simulink subsystem "linear_slope_score"  (R2020b)
settings: Solver=VariableStepAuto  StartTime=0.0  StopTime=10.0  RelTol=1e-3
settings Model: Creator=RH  LastModifiedBy=Marco

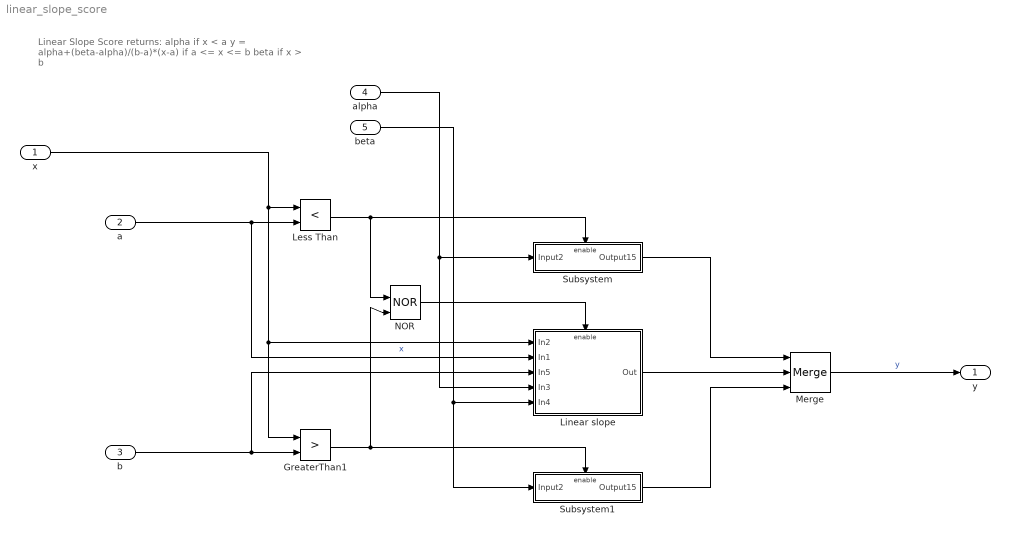
== system linear_slope_score ==
  note: Linear Slope Score
      | returns:
      |
      | alpha if x < a
      | y = alpha+(beta-alpha)/(b-a)*(x-a) if a <= x <= b
      | beta if x > b
  x : Inport
  a : Inport  Port=2
  b : Inport  Port=3
  alpha : Inport  Port=4
  beta : Inport  Port=5
  GreaterThan1 : RelationalOperator  Operator=>  OutDataTypeStr=boolean  RndMeth=Simplest
  Less Than : RelationalOperator  Operator=<  OutDataTypeStr=boolean  RndMeth=Simplest
  Linear slope : Subsystem
  Merge : Merge  Inputs=3
  NOR : Logic  Operator=NOR  IconShape=distinctive  AllPortsSameDT=off  OutDataTypeStr=boolean
  Subsystem : Subsystem
  Subsystem1 : Subsystem
  y : Outport
  wires:
  b/1 -> Linear slope/3(In5), GreaterThan1/2
  Less Than/1 -> NOR/1, Subsystem/Enable
  x/1 -> Linear slope/1(In2), GreaterThan1/1, Less Than/1  "x"
  beta/1 -> Linear slope/5(In4), Subsystem1/1(Input2)
  alpha/1 -> Subsystem/1(Input2), Linear slope/4(In3)
  Subsystem/1(Output15) -> Merge/1
  GreaterThan1/1 -> NOR/2, Subsystem1/Enable
  a/1 -> Linear slope/2(In1), Less Than/2
  NOR/1 -> Linear slope/Enable
  Subsystem1/1(Output15) -> Merge/3
  Linear slope/1(Out) -> Merge/2
  Merge/1 -> y/1  "y"

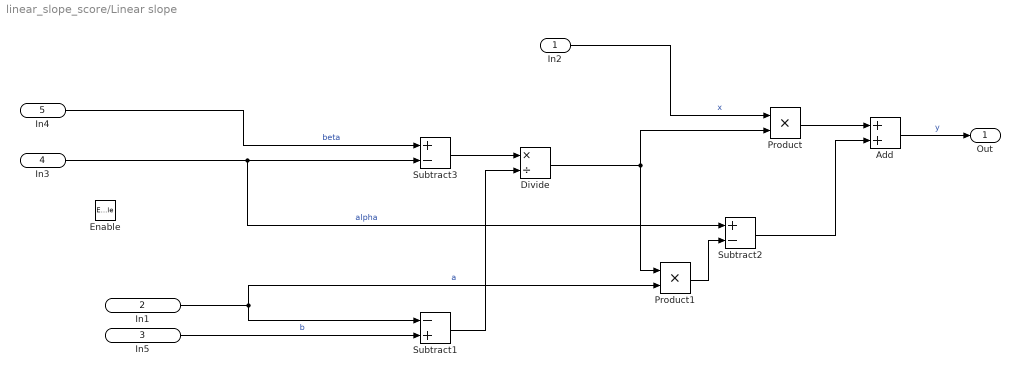
== system linear_slope_score/Linear slope ==
  In2 : Inport
  In1 : Inport  Port=2
  In5 : Inport  Port=3
  In3 : Inport  Port=4  Unit=1
  In4 : Inport  Port=5  Unit=1
  Enable : EnablePort
  Add : Sum
  Divide : Product  Inputs=*/
  Product : Product
  Product1 : Product
  Subtract1 : Sum  Inputs=-+
  Subtract2 : Sum  Inputs=+-
  Subtract3 : Sum  Inputs=+-
  Out : Outport  Unit=1
  wires:
  In4/1 -> Subtract3/1  "beta"
  Subtract2/1 -> Add/2
  Product1/1 -> Subtract2/2
  Add/1 -> Out/1  "y"
  Product/1 -> Add/1
  Divide/1 -> Product1/1, Product/2
  Subtract1/1 -> Divide/2
  In5/1 -> Subtract1/2  "b"
  In1/1 -> Subtract1/1, Product1/2  "a"
  Subtract3/1 -> Divide/1
  In2/1 -> Product/1  "x"
  In3/1 -> Subtract3/2, Subtract2/1  "alpha"

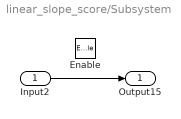
== system linear_slope_score/Subsystem ==
  Input2 : Inport
  Enable : EnablePort
  Output15 : Outport
  wires:
  Input2/1 -> Output15/1

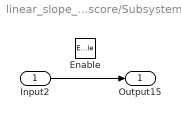
== system linear_slope_score/Subsystem1 ==
  Input2 : Inport
  Enable : EnablePort
  Output15 : Outport
  wires:
  Input2/1 -> Output15/1
